simulink model "Plant_Model"  (R2024b)
settings: Solver=VariableStepAuto  StartTime=0.0  StopTime=10  RelTol=1e-3
values from neighbouring files (symbols this model uses):
  A = 2    [parameters.m]
  c1 = 0.86    [parameters.m]
  c2 = 33.82    [parameters.m]
  c3 = 0.36    [parameters.m]
  Cw = 0.3    [parameters.m]
  g = 9.81    [parameters.m]
  JR = 0.8    [parameters.m]
  m = 1500    [parameters.m]
  rho = 1.2    [parameters.m]
  rR = 0.3    [parameters.m]
  vf_0 = 100    [parameters.m]
settings Model: Creator=devap  LastModifiedBy=devap
settings DebuggingCC: UnderSpecifiedDimensionMsg=warning

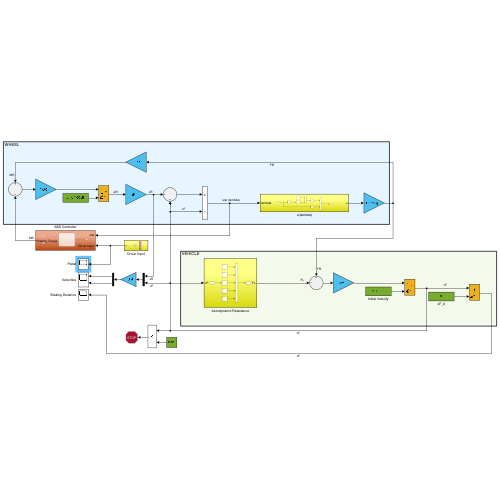
[thumbnail: Simulink's stored preview of the top-level diagram]
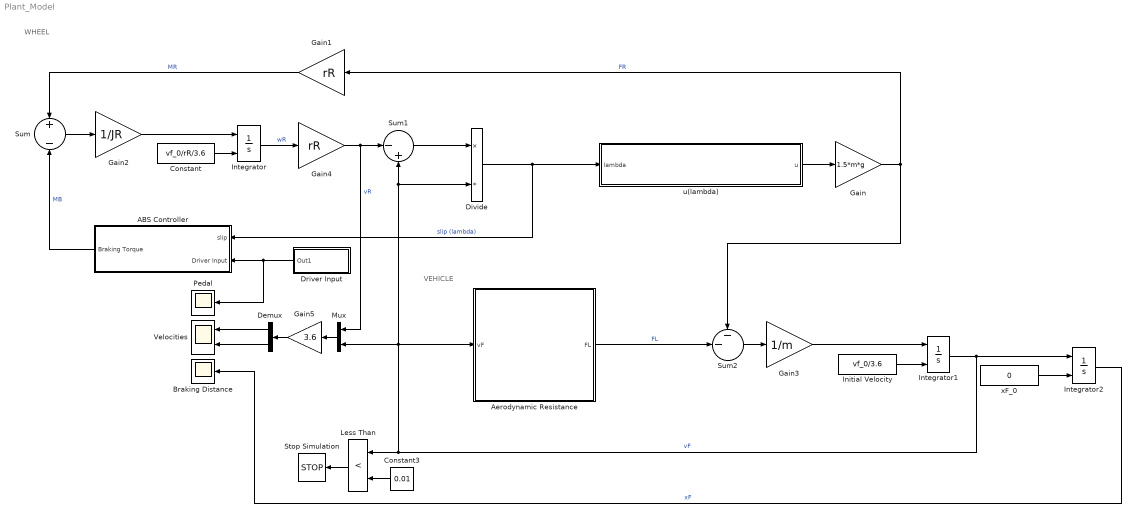
== system Plant_Model ==
  note: WHEEL
  note: VEHICLE
  ABS Controller : Subsystem
  Aerodynamic Resistance : Subsystem
  Braking Distance : Scope
  Constant : Constant  Value=vf_0/rR/3.6
  Constant3 : Constant  Value=0.01
  Demux : Demux  Outputs=2
  Divide : Product  Inputs=*/
  Driver Input : Subsystem
  Gain : Gain  Gain=1.5*m*g
  Gain1 : Gain  Gain=rR
  Gain2 : Gain  Gain=1/JR
  Gain3 : Gain  Gain=1/m
  Gain4 : Gain  Gain=rR
  Gain5 : Gain  Gain=3.6
  Initial Velocity : Constant  Value=vf_0/3.6
  Integrator : Integrator  InitialConditionSource=external  LimitOutput=on  LowerSaturationLimit=0
  Integrator1 : Integrator  InitialConditionSource=external  LimitOutput=on  LowerSaturationLimit=0
  Integrator2 : Integrator  InitialConditionSource=external  LowerSaturationLimit=0
  Less Than : RelationalOperator  Operator=<  OutDataTypeStr=boolean  RndMeth=Simplest  InputSameDT=off
  Mux : Mux  Inputs=2
  Pedal : Scope
  Stop Simulation : Stop
  Sum : Sum  Inputs=+|-
  Sum1 : Sum  Inputs=|-+
  Sum2 : Sum  Inputs=--|
  Velocities : Scope  NumInputPorts=2
  u(lambda) : Subsystem
  xF_0 : Constant  Value=0
  wires:
  u(lambda)/1(u) -> Gain/1
  Gain1/1 -> Sum/1  "MR"
  Gain/1 -> Gain1/1, Sum2/1  "FR"
  Sum/1 -> Gain2/1
  Gain2/1 -> Integrator/1
  Constant/1 -> Integrator/2
  Integrator/1 -> Gain4/1  "wR"
  Gain4/1 -> Mux/1, Sum1/1  "vR"
  Sum1/1 -> Divide/1
  Divide/1 -> u(lambda)/1(lambda), ABS Controller/1(slip)  "slip (lambda)"
  Aerodynamic Resistance/1(FL) -> Sum2/2  "FL"
  Sum2/1 -> Gain3/1
  Gain3/1 -> Integrator1/1
  Initial Velocity/1 -> Integrator1/2
  Integrator1/1 -> Mux/2, Divide/2, Sum1/2, Aerodynamic Resistance/1(vF), Less Than/1, Integrator2/1  "vF"
  xF_0/1 -> Integrator2/2
  Integrator2/1 -> Braking Distance/1  "xF"
  Less Than/1 -> Stop Simulation/1
  Constant3/1 -> Less Than/2
  Driver Input/1(Out1) -> Pedal/1, ABS Controller/2(Driver Input)
  ABS Controller/1(Braking Torque) -> Sum/2  "MB"
  Demux/1 -> Velocities/1
  Demux/2 -> Velocities/2
  Mux/1 -> Gain5/1
  Gain5/1 -> Demux/1

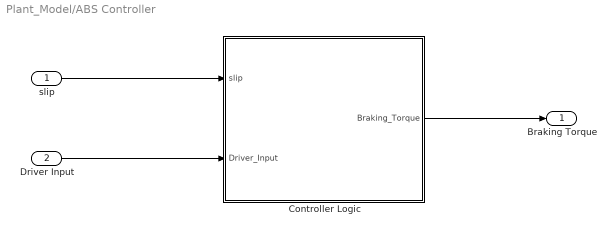
== system Plant_Model/ABS Controller ==
  slip : Inport
  Driver Input : Inport  Port=2
  Controller Logic : Stateflow chart  TreatAsAtomicUnit=on
      settings: PortSchema="{\"entries\":[{\"content\":{\"sides\":[{\"content\":{},\"type\":\"ConnectorPlacement.EquallySpacedRectSide\",\"uuid\":\"21f18844-d46f-4192-8888-e19f26fc3edc\"},{\"content\":{\"side\":\"RIGHT\"},\"type\":\"ConnectorPlacement.EquallySpacedRectSide\",\"uuid\":\"7bd71700-bad4-4cbb-9483-04161d3aff77\"},{\"content\":{\"connectorIds\":[\"In2\",\"In1\"],\"side\":\"TOP\"},\"type\":\"ConnectorPlacement.EquallySpacedRectSide\",\"uuid\":\"4756a897-bcf0-41d1-bf8d-a96ee74f6ad2\"},{\"content\":{\"connectorIds\":[\"Out1\"],\"side\":\"BOTTOM\"},\"type\":\"ConnectorPlacement.EquallySpacedRectSide\",\"uuid\":\"313fe5f9-b121-4e9c-8752-7e0554df123c\"}]},\"type\":\"ConnectorPlacement.EquallySpacedConnector\",\"uuid\":\"67e74c9c-ac74-4bfd-968a-12aff3b01f59\"}],\"packageUris\":[\"http://schema.mathworks.com/mf0/Connector/R2020b\"],\"version\":\"1.0\"}"
  Braking Torque : Outport
  wires:
  slip/1 -> Controller Logic/1(slip)
  Controller Logic/1(Braking_Torque) -> Braking Torque/1
  Driver Input/1 -> Controller Logic/2(Driver_Input)

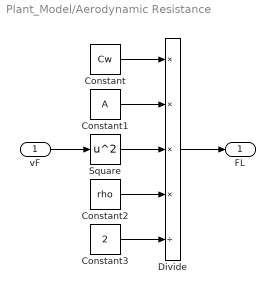
== system Plant_Model/Aerodynamic Resistance ==
  vF : Inport
  Constant : Constant  Value=Cw
  Constant1 : Constant  Value=A
  Constant2 : Constant  Value=rho
  Constant3 : Constant  Value=2
  Divide : Product  Inputs=****/
  Square : Math  Operator=square
  FL : Outport
  wires:
  Divide/1 -> FL/1
  vF/1 -> Square/1
  Square/1 -> Divide/3
  Constant/1 -> Divide/1
  Constant1/1 -> Divide/2
  Constant2/1 -> Divide/4
  Constant3/1 -> Divide/5

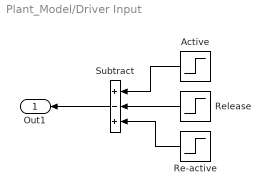
== system Plant_Model/Driver Input ==
  Active : Step  SampleTime=0
  Re-active : Step  Time=3  SampleTime=0
  Release : Step  Time=2  SampleTime=0
  Subtract : Sum  Inputs=+-+
  Out1 : Outport
  wires:
  Active/1 -> Subtract/1
  Release/1 -> Subtract/2
  Subtract/1 -> Out1/1
  Re-active/1 -> Subtract/3

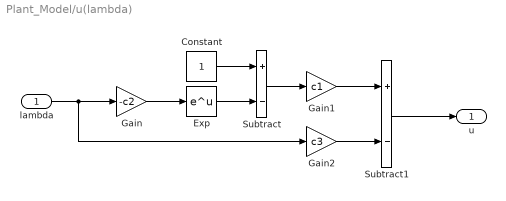
== system Plant_Model/u(lambda) ==
  lambda : Inport
  Constant : Constant
  Exp : Math
  Gain : Gain  Gain=-c2
  Gain1 : Gain  Gain=c1
  Gain2 : Gain  Gain=c3
  Subtract : Sum  Inputs=+-
  Subtract1 : Sum  Inputs=+-
  u : Outport
  wires:
  lambda/1 -> Gain2/1, Gain/1
  Gain/1 -> Exp/1
  Exp/1 -> Subtract/2
  Constant/1 -> Subtract/1
  Subtract/1 -> Gain1/1
  Gain1/1 -> Subtract1/1
  Gain2/1 -> Subtract1/2
  Subtract1/1 -> u/1

== stateflow chart Plant_Model/ABS Controller/Controller Logic ==
  state Braking_Input
    state Delay
      during: Braking_Torque=0;
    state Braking
      during: Braking_Torque=BT_max;
    (default) -> Delay
    Delay -> Braking : [after(1,sec) && Driver_Input == 1]
  state ABS_ON
    during: Braking_Torque=0;
  state ABS_OFF
    during: Braking_Torque=BT_max;
  (default) -> Braking_Input
  Braking_Input -> ABS_ON : [Driver_Input == 1 && slip > 0.13]
  ABS_OFF -> ABS_ON [order 1] : [Driver_Input == 1 && slip > 0.13]
  ABS_ON -> ABS_OFF : [Driver_Input == 1 && slip <= 0.13]
  ABS_OFF -> Braking_Input [order 2] : [Driver_Input == 0]
  data: slip input; Driver_Input input; Braking_Torque output; BT_max parameter
